simulink model "lab9_10dsa"  (R2024a)
settings: Solver=VariableStepAuto  StartTime=0.0  StopTime=10.0  RelTol=1e-3
model workspace (MAT data in the model file):
  test = 'lab9_10_my.fis'
libraries: fuzblock x1
settings Model: Creator=Ivan  LastModifiedBy=Ivan

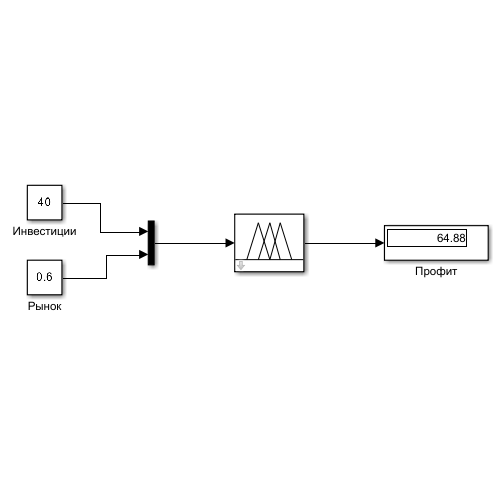
[thumbnail: Simulink's stored preview of the top-level diagram]
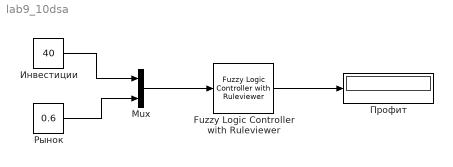
== system lab9_10dsa ==
  Fuzzy Logic Controller with Ruleviewer : fuzblock/Fuzzy Logic  Controller  with Ruleviewer  fismatrix=lab9_10_my  Ts=2
  Mux : Mux  Inputs=2
  Инвестиции : Constant  Value=40
  Профит : Display
  Рынок : Constant  Value=0.6
  wires:
  Fuzzy Logic Controller with Ruleviewer/1 -> Профит/1
  Mux/1 -> Fuzzy Logic Controller with Ruleviewer/1
  Инвестиции/1 -> Mux/1
  Рынок/1 -> Mux/2
